simulink model "terrainfollow_revised"  (R2018a)
settings: Solver=VariableStepAuto  StartTime=0.0  StopTime=60  FixedStep=0.00001  RelTol=1e-3
values from neighbouring files (symbols this model uses):
  A = [0 0 0.00013165266625 3.15369085605e-06 -1.52707114267e-20 299.999999993 0 -32.1699999992 -6.02299064272e-14 0 0 0 ... (25 elements, 5x5)]    [redu_ss_terrainfollow.mat]    (also in reducefun_terrainfollow.m = A_longitude_lo(1:5,1:5))
  B = [0  0; 0  0; 0.00154396044469  -0.00453382204302; -9.49308816068e-07  -0.00111635553349; 0  -0.0570163434913]    [redu_ss_terrainfollow.mat]    (also in reducefun_terrainfollow.m = A_longitude_lo(1:5,[6 7]))
  C = [1 0 0 0 0 0 1 0 0 0 0 0 ... (25 elements, 5x5)]    [redu_ss_terrainfollow.mat]    (also in reducefun_terrainfollow.m = eye(5))
  D = [0  0; 0  0; 0  0; 0  0; 0  0]    [redu_ss_terrainfollow.mat]    (also in reducefun_terrainfollow.m = zeros(5,2))
  ele_lowlim = -25    - de0    [terrainfollow_run.m]    (also in terrainfollow_sim_bigcanyon.m)
  ele_uplim = 25     - de0    [terrainfollow_run.m]    (also in terrainfollow_sim_bigcanyon.m)
  gclear = 40    [terrainfollow_run.m]    (also in terrainfollow_sim_bigcanyon.m)
  h0 = 1500    [terrainfollow_run.m]    (also in terrainfollow_sim_bigcanyon.m)
  K_i = K_f(:,2:5)    [terrainfollow_run.m]    (also in terrainfollow_sim_bigcanyon.m)
  K_o = K_f(:,1)    [terrainfollow_run.m]    (also in terrainfollow_sim_bigcanyon.m)
  th_lowlim = 1000   - th0    [terrainfollow_run.m]    (also in terrainfollow_sim_bigcanyon.m)
  th_uplim = 19000  - th0    [terrainfollow_run.m]    (also in terrainfollow_sim_bigcanyon.m)
  v0 = ft2m*trim_state_lo(7)    [terrainfollow_run.m]    (also in terrainfollow_sim_bigcanyon.m)
libraries: aerolibconvert2 x5
settings Model: Creator=Lukas  LastModifiedBy=Lukas
settings CodeAppCC: StateflowObjectComments=on

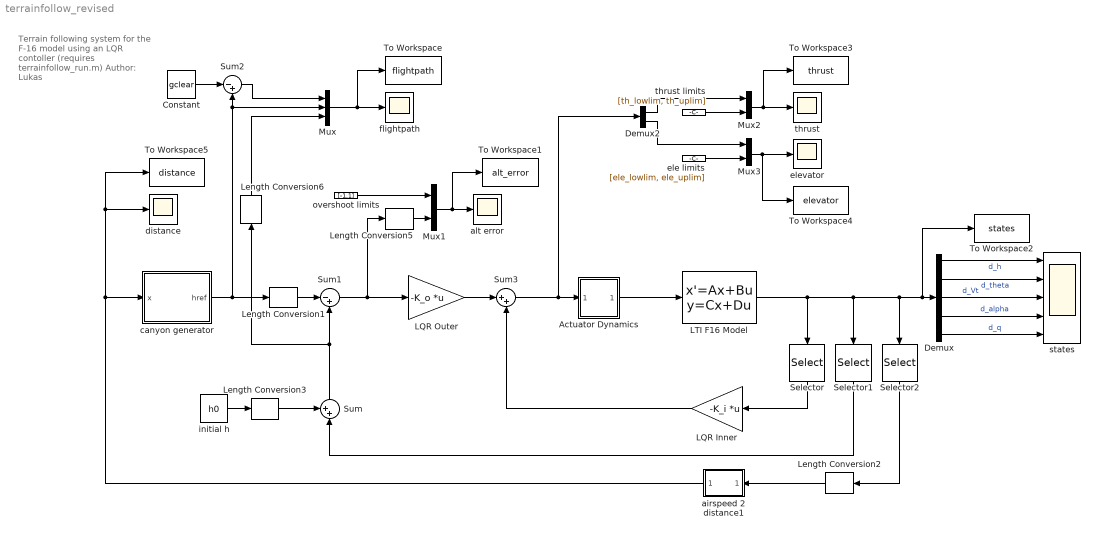
== system terrainfollow_revised ==
  note: Terrain following system for
      | the F-16 model using an LQR
      | contoller
      |
      | (requires terrainfollow_run.m)
      |
      | Author: Lukas
  Actuator Dynamics : Subsystem
  Constant : Constant  Value=gclear
  Demux : Demux  Outputs=5
  Demux2 : Demux  Outputs=2
  LQR Inner : Gain  Gain=-K_i  Multiplication=Matrix(K*u)  SaturateOnIntegerOverflow=on  OutDataTypeStr=Inherit: Same as input  ParamDataTypeStr=Inherit: Same as input
  LQR Outer : Gain  Gain=-K_o  Multiplication=Matrix(K*u)  SaturateOnIntegerOverflow=on  OutDataTypeStr=Inherit: Same as input  ParamDataTypeStr=Inherit: Same as input
  "LTI F16 Model " : StateSpace  A=A  B=B  C=C  D=D  InitialCondition=0
      mask Display: image('f16thumb.jpg');
  Length Conversion1 : aerolibconvert2/Length Conversion  IU=m  OU=ft
  Length Conversion2 : aerolibconvert2/Length Conversion  IU=ft  OU=m
  Length Conversion3 : aerolibconvert2/Length Conversion  IU=m  OU=ft
  Length Conversion5 : aerolibconvert2/Length Conversion  IU=ft  OU=m
  Length Conversion6 : aerolibconvert2/Length Conversion  IU=ft  OU=m
  Mux : Mux  Inputs=3
  Mux1 : Mux  Inputs=2
  Mux2 : Mux  Inputs=2
  Mux3 : Mux  Inputs=2
  Selector : Selector  InputPortWidth=5  IndexOptions=Index vector (dialog)  Indices=[2 3 4 5]  OutputSizes=1
  Selector1 : Selector  InputPortWidth=5  IndexOptions=Index vector (dialog)  Indices=1  OutputSizes=1
  Selector2 : Selector  InputPortWidth=5  IndexOptions=Index vector (dialog)  Indices=[2 3 4]  OutputSizes=1
  Sum : Sum  Inputs=++|
  Sum1 : Sum  Inputs=|-+
  Sum2 : Sum  Inputs=|-+
  Sum3 : Sum  Inputs=|++
  To Workspace : ToWorkspace  VariableName=flightpath  SaveFormat=Timeseries  SampleTime=-1
  To Workspace1 : ToWorkspace  VariableName=alt_error  SaveFormat=Timeseries  SampleTime=-1
  To Workspace2 : ToWorkspace  VariableName=states  SaveFormat=Timeseries  SampleTime=-1
  To Workspace3 : ToWorkspace  VariableName=thrust  SaveFormat=Timeseries  SampleTime=-1
  To Workspace4 : ToWorkspace  VariableName=elevator  SaveFormat=Timeseries  SampleTime=-1
  To Workspace5 : ToWorkspace  VariableName=distance  SaveFormat=Timeseries  SampleTime=-1
  airspeed 2 distance1 : Subsystem
  alt error : Scope
  canyon generator : Subsystem
      mask Display: image(imread('canyon.jpg'))
  distance : Scope
  ele limits : Constant  Value=[ele_lowlim, ele_uplim]
  elevator : Scope
  flightpath : Scope
  initial h : Constant  Value=h0
  overshoot limits : Constant  Value=[-1,1]
  states : Scope  NumInputPorts=5
  thrust : Scope
  thrust limits : Constant  Value=[th_lowlim, th_uplim]
  wires:
  Selector/1 -> LQR Inner/1
  LQR Inner/1 -> Sum3/2
  "LTI F16 Model "/1 -> Selector/1, Selector1/1, Selector2/1, To Workspace2/1, Demux/1
  Sum3/1 -> Demux2/1, Actuator Dynamics/1(In1)
  Demux/1 -> states/1  "d_h"
  Demux/2 -> states/2  "d_theta"
  Demux/4 -> states/4  "d_alpha"
  Demux/5 -> states/5  "d_q"
  canyon generator/1(href) -> Mux/2, Sum2/2, Length Conversion1/1
  airspeed 2 distance1/1(Out1) -> canyon generator/1(x), distance/1, To Workspace5/1
  LQR Outer/1 -> Sum3/1
  initial h/1 -> Length Conversion3/1
  Length Conversion3/1 -> Sum/1
  Length Conversion1/1 -> Sum1/1
  Sum1/1 -> Length Conversion5/1, LQR Outer/1
  Sum/1 -> Length Conversion6/1, Sum1/2
  Demux/3 -> states/3  "d_Vt"
  ele limits/1 -> Mux3/2
  Demux2/2 -> Mux3/1
  thrust limits/1 -> Mux2/2
  Demux2/1 -> Mux2/1
  Actuator Dynamics/1(Out1) -> "LTI F16 Model "/1
  overshoot limits/1 -> Mux1/1
  Length Conversion6/1 -> Mux/3
  Length Conversion5/1 -> Mux1/2
  Sum2/1 -> Mux/1
  Constant/1 -> Sum2/1
  Mux/1 -> To Workspace/1, flightpath/1
  Mux1/1 -> To Workspace1/1, alt error/1
  Mux2/1 -> thrust/1, To Workspace3/1
  Mux3/1 -> elevator/1, To Workspace4/1
  Selector2/1 -> Length Conversion2/1
  Selector1/1 -> Sum/2
  Length Conversion2/1 -> airspeed 2 distance1/1(In1)

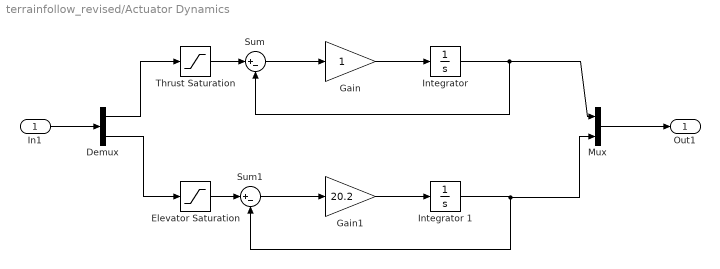
== system terrainfollow_revised/Actuator Dynamics ==
  In1 : Inport
  Demux : Demux  Outputs=2
  Elevator Saturation : Saturate  UpperLimit=ele_uplim  LowerLimit=ele_lowlim
  Gain : Gain  SaturateOnIntegerOverflow=on  OutDataTypeStr=Inherit: Same as input  ParamDataTypeStr=Inherit: Same as input
  Gain1 : Gain  Gain=20.2  SaturateOnIntegerOverflow=on  OutDataTypeStr=Inherit: Same as input  ParamDataTypeStr=Inherit: Same as input
  "Integrator " : Integrator  UpperSaturationLimit=30  LowerSaturationLimit=-30
  Integrator 1 : Integrator  UpperSaturationLimit=25  LowerSaturationLimit=-25
  Mux : Mux  Inputs=2
  Sum : Sum  Inputs=|+-  SaturateOnIntegerOverflow=on  InputSameDT=on  OutDataTypeStr=Inherit: Same as first input
  Sum1 : Sum  Inputs=|+-  SaturateOnIntegerOverflow=on  InputSameDT=on  OutDataTypeStr=Inherit: Same as first input
  Thrust Saturation : Saturate  UpperLimit=th_uplim  LowerLimit=th_lowlim
  Out1 : Outport
  wires:
  Mux/1 -> Out1/1
  In1/1 -> Demux/1
  Sum1/1 -> Gain1/1
  Gain1/1 -> Integrator 1/1
  Integrator 1/1 -> Mux/2, Sum1/2
  Sum/1 -> Gain/1
  "Integrator "/1 -> Mux/1, Sum/2
  Gain/1 -> "Integrator "/1
  Demux/1 -> Thrust Saturation/1
  Demux/2 -> Elevator Saturation/1
  Thrust Saturation/1 -> Sum/1
  Elevator Saturation/1 -> Sum1/1

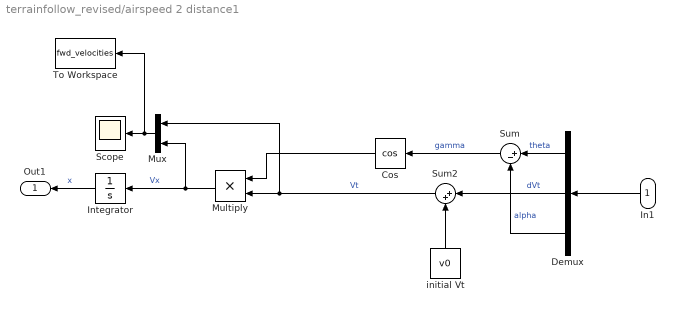
== system terrainfollow_revised/airspeed 2 distance1 ==
  In1 : Inport
  Cos : Trigonometry  Operator=cos
  Demux : Demux  Outputs=3
  Integrator : Integrator
  Multiply : Product
  Mux : Mux  Inputs=2
  Scope : Scope
  Sum : Sum  Inputs=|+-
  Sum2 : Sum  Inputs=|++
  To Workspace : ToWorkspace  VariableName=fwd_velocities  SaveFormat=Timeseries  SampleTime=-1
  initial Vt : Constant  Value=v0
  Out1 : Outport
  wires:
  Integrator/1 -> Out1/1  "x"
  In1/1 -> Demux/1
  initial Vt/1 -> Sum2/2
  Demux/2 -> Sum2/1  "dVt"
  Demux/1 -> Sum/1  "theta"
  Demux/3 -> Sum/2  "alpha"
  Sum/1 -> Cos/1  "gamma"
  Sum2/1 -> Mux/1, Multiply/2  "Vt"
  Cos/1 -> Multiply/1
  Multiply/1 -> Mux/2, Integrator/1  "Vx"
  Mux/1 -> To Workspace/1, Scope/1

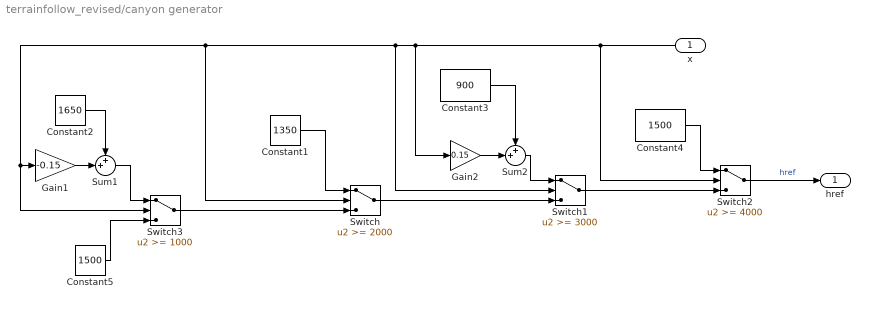
== system terrainfollow_revised/canyon generator ==
  x : Inport
  Constant1 : Constant  Value=1350
  Constant2 : Constant  Value=1650
  Constant3 : Constant  Value=900
  Constant4 : Constant  Value=1500
  Constant5 : Constant  Value=1500
  Gain1 : Gain  Gain=-0.15
  Gain2 : Gain  Gain=0.15
  Sum1 : Sum  Inputs=++|
  Sum2 : Sum  Inputs=++|
  Switch : Switch  Threshold=2000  ZeroCross=off
  Switch1 : Switch  Threshold=3000  ZeroCross=off
  Switch2 : Switch  Threshold=4000  ZeroCross=off
  Switch3 : Switch  Threshold=1000  ZeroCross=off
  href : Outport
  wires:
  Constant1/1 -> Switch/1
  x/1 -> Switch2/2, Gain2/1, Switch1/2, Switch/2, Gain1/1, Switch3/2
  Switch/1 -> Switch1/3
  Gain2/1 -> Sum2/2
  Constant3/1 -> Sum2/1
  Sum2/1 -> Switch1/1
  Switch1/1 -> Switch2/3
  Constant4/1 -> Switch2/1
  Switch2/1 -> href/1  "href"
  Switch3/1 -> Switch/3
  Constant5/1 -> Switch3/3
  Sum1/1 -> Switch3/1
  Gain1/1 -> Sum1/2
  Constant2/1 -> Sum1/1
